simulink model "IP02_FreqTest"  (R2024b)
settings: Solver=ode45  StartTime=0.0  StopTime=120  RelTol=1e-3
undefined symbols (not defined in the file): A_cart, B_cart, C_cart, D_cart, K_a, V_sat
settings Model: Creator=Karim Negm  LastModifiedBy=Karim Negm

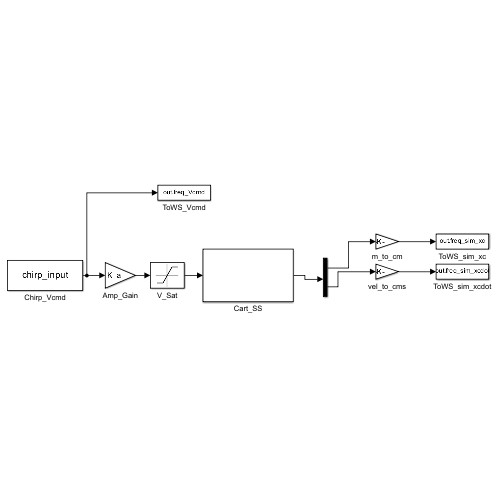
[thumbnail: Simulink's stored preview of the top-level diagram]
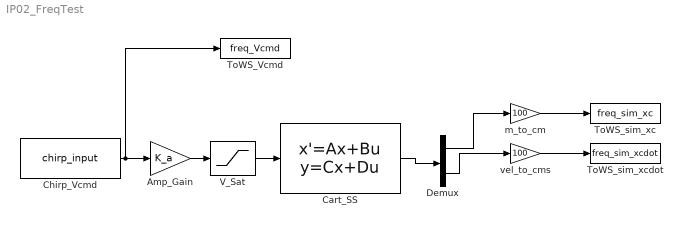
== system IP02_FreqTest ==
  Amp_Gain : Gain  Gain=K_a
  Cart_SS : StateSpace  A=A_cart  B=B_cart  C=C_cart  D=D_cart  InitialCondition=0
  Chirp_Vcmd : FromWorkspace  VariableName=chirp_input
  Demux : Demux  Outputs=2
  ToWS_Vcmd : ToWorkspace  VariableName=freq_Vcmd  SaveFormat=Timeseries  SampleTime=-1
  ToWS_sim_xc : ToWorkspace  VariableName=freq_sim_xc  SaveFormat=Timeseries  SampleTime=-1
  ToWS_sim_xcdot : ToWorkspace  VariableName=freq_sim_xcdot  SaveFormat=Timeseries  SampleTime=-1
  V_Sat : Saturate  UpperLimit=V_sat  LowerLimit=-V_sat
  m_to_cm : Gain  Gain=100
  vel_to_cms : Gain  Gain=100
  wires:
  Chirp_Vcmd/1 -> Amp_Gain/1, ToWS_Vcmd/1
  Amp_Gain/1 -> V_Sat/1
  V_Sat/1 -> Cart_SS/1
  Cart_SS/1 -> Demux/1
  Demux/1 -> m_to_cm/1
  Demux/2 -> vel_to_cms/1
  m_to_cm/1 -> ToWS_sim_xc/1
  vel_to_cms/1 -> ToWS_sim_xcdot/1
